simulink model "acceleration_model"  (R2019b)
settings: Solver=VariableStepAuto  StartTime=0.0  StopTime=30.0  RelTol=1e-9
undefined symbols (not defined in the file): P, x0, x0_dot
settings Model: Creator=Charlie  LastModifiedBy=Charlie

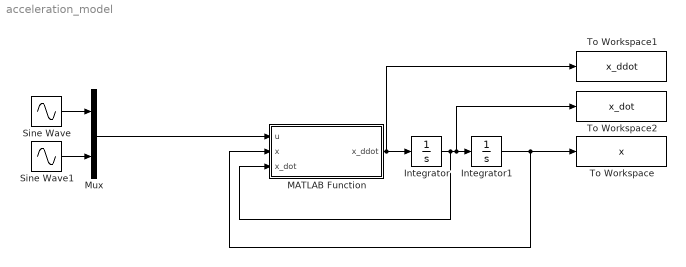
== system acceleration_model ==
  Integrator : Integrator  InitialCondition=x0_dot
  Integrator1 : Integrator  InitialCondition=x0
  MATLAB Function : MATLAB Function  TreatAsAtomicUnit=on
  Mux : Mux  Inputs=2
  Sine Wave : Sin  Amplitude=-P.amp*P.frq^2  Frequency=P.frq  Phase=-pi/2  SampleTime=0
  Sine Wave1 : Sin  Amplitude=-P.amp*P.frq^2  Frequency=P.frq  SampleTime=0
  To Workspace : ToWorkspace  VariableName=x  SampleTime=-1
  To Workspace1 : ToWorkspace  VariableName=x_ddot  SampleTime=-1
  To Workspace2 : ToWorkspace  VariableName=x_dot  SampleTime=-1
  wires:
  MATLAB Function/1(x_ddot) -> To Workspace1/1, Integrator/1
  Integrator/1 -> MATLAB Function/3(x_dot), To Workspace2/1, Integrator1/1
  Sine Wave/1 -> Mux/1
  Sine Wave1/1 -> Mux/2
  Integrator1/1 -> MATLAB Function/2(x), To Workspace/1
  Mux/1 -> MATLAB Function/1(u)

== matlab function acceleration_model/MATLAB Function ==
  data: u input; x_ddot output; x input; x_dot input; P parameter
function x_ddot = EOM(u, x, x_dot, P)

theta     = x(1:2);
phi       = x(3:4);

theta_dot = x_dot(1:2);
phi_dot   = x_dot(3:4);

M = zeros(10);
M_dot = zeros(10);
b_dot = zeros(10,1);
% Row 1
M(1,4) = P.a4*sin(phi(2)) - P.c4*cos(phi(2));
M(1,5) = 1;
% Row 2
M(2,1) =-P.r2*sin(theta(1));
M(2,3) =-P.a4*cos(phi(1))*sin(phi(2)) + P.c4*cos(phi(1))*cos(phi(2));
M(2,4) =-P.a4*sin(phi(1))*cos(phi(2)) - P.c4*cos(phi(1))*sin(phi(2));
M(2,6) = 1;
% Row 3
M(3,1) = P.r2*cos(theta(1));
M(3,3) =-P.a4*sin(phi(1))*sin(phi(2)) + P.c4*sin(phi(1))*cos(phi(2));
M(3,4) = P.a4*cos(phi(1))*cos(phi(2)) + P.c4*cos(phi(1))*sin(phi(2));
M(3,7) = 1;
% Row 4
M(4,5) = x(5);
M(4,6) = x(6);
M(4,7) = x(7);
% Row 5
M(5,2) = P.r6*sin(theta(2));
M(5,4) =-P.c8*cos(phi(2));
M(5,8) = 1;
% Row 6
M(6,3) = P.b8*sin(phi(1)) + P.c8*cos(phi(1))*cos(phi(2));
M(6,4) =-P.c8*sin(phi(1))*sin(phi(2));
M(6,9) = 1;
% Row 7
M(7,2) = P.r6*cos(theta(2));
M(7,3)  =-P.b8*cos(phi(1)) + P.c8*sin(phi(1))*cos(phi(2));
M(7,4)  = P.c8*cos(phi(1))*sin(phi(2));
M(7,10) = 1;
% Row 8
M(8,8)  = x(8);
M(8,9)  = x(9);
M(8,10) = x(10);
% Row 9
M(9,1) = 1;
% Row 10
M(10,2) = 1;
%
%
%
%
% Row 1
M_dot(1,4) = phi_dot(2)*(P.a4*cos(phi(2))+P.c4*sin(phi(2)));
% Row 2
M_dot(2,1) =-theta_dot(1)*P.r2*cos(theta(1));
M_dot(2,3) = phi_dot(1)*( P.a4*sin(phi(1))*sin(phi(2)) - P.c4*sin(phi(1))*cos(phi(2))) ...
           - phi_dot(2)*( P.a4*cos(phi(1))*cos(phi(2)) + P.c4*cos(phi(1))*sin(phi(2)));
M_dot(2,4) = phi_dot(1)*(-P.a4*cos(phi(1))*cos(phi(2)) + P.c4*sin(phi(1))*sin(phi(2))) ...
           + phi_dot(2)*( P.a4*sin(phi(1))*sin(phi(2)) - P.c4*cos(phi(1))*cos(phi(2)));
% Row 3
M_dot(3,1) =-theta_dot(1)*P.r2*sin(theta(1));
M_dot(3,3) = phi_dot(1)*(-P.a4*cos(phi(1))*sin(phi(2)) + P.c4*cos(phi(1))*cos(phi(2))) ...
           + phi_dot(2)*(-P.a4*sin(phi(1))*cos(phi(2)) - P.c4*sin(phi(1))*sin(phi(2)));
M_dot(3,4) = phi_dot(1)*(-P.a4*sin(phi(1))*cos(phi(2)) - P.c4*sin(phi(1))*sin(phi(2))) ...
           + phi_dot(2)*(-P.a4*cos(phi(1))*sin(phi(2)) + P.c4*cos(phi(1))*cos(phi(2)));
% Row 4
M_dot(4,5) = x_dot(5);
M_dot(4,6) = x_dot(6);
M_dot(4,7) = x_dot(7);
% Row 5
M_dot(5,2) = theta_dot(2)*P.r6*cos(theta(2));
M_dot(5,4) = phi_dot(2)*P.c8*sin(phi(2));
% Row 6
M_dot(6,3) = phi_dot(1)*(P.b8*cos(phi(1))-P.c8*sin(phi(1))*cos(phi(2))) ...
           - phi_dot(2)*P.c8*cos(phi(1))*sin(phi(2));
M_dot(6,4) =-phi_dot(1)*P.c8*cos(phi(1))*sin(phi(2)) ...
           - phi_dot(2)*P.c8*sin(phi(1))*cos(phi(2));
% Row 7
M_dot(7,2) =-theta_dot(2)*P.r6*sin(theta(2));
M_dot(7,3) = phi_dot(1)*(P.b8*sin(phi(1))+P.c8*cos(phi(1))*cos(phi(2))) ...
           - phi_dot(2)*P.c8*sin(phi(1))*sin(phi(2));
M_dot(7,4) =-phi_dot(1)*P.c8*sin(phi(1))*sin(phi(2)) ...
           + phi_dot(2)*P.c8*cos(phi(1))*cos(phi(2));
% Row 8
M_dot(8,8) = x_dot(8);
M_dot(8,9) = x_dot(9);
M_dot(8,10) = x_dot(10);
% Row 9
b_dot(9)=u(1);
% Row 10
b_dot(10)=u(2);
%
x_ddot = M\(b_dot-M_dot*x_dot);
end
